simulink model "untitled1"  (R2025a)
settings: Solver=VariableStepAuto  StartTime=0.0  StopTime=5  RelTol=1e-3
libraries: spsControlledVoltageSourceLib x2, spsStepperMotorLib x1, spspowerguiLib x1
settings Model: Creator=One  LastModifiedBy=One

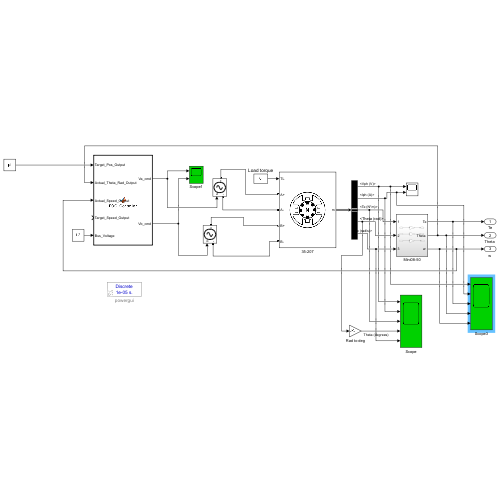
[thumbnail: Simulink's stored preview of the top-level diagram]
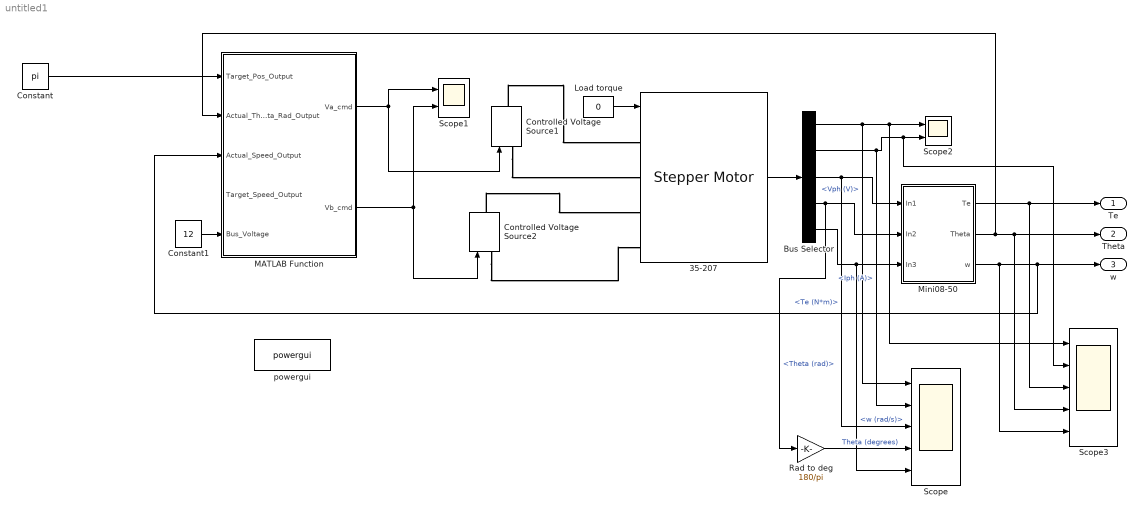
== system untitled1 ==
  35-207 : spsStepperMotorLib/Stepper Motor  MotorType=Permanent-magnet / Hybrid  NumberOfPhases_1=2  NumberOfPhases_2=3  PresetModel_1=<empty>  PresetModel_2=<empty>  L=5.44e-3  Lmax=10e-3  Lmin=2e-3  R=4.85  Step_angle=1.8  Psim=4.35e-3  Tdm=0.06  J=1e-6  B=1e-7*1000  w0=0  pos0=0  TsPowergui=0  TsBlock=-1
  Bus Selector : BusSelector  OutputSignals=Vph (V),Iph (A),Te (N*m),Theta (rad),w (rad/s)
  Constant : Constant  Value=pi
  Constant1 : Constant  Value=12
  Controlled Voltage Source1 : spsControlledVoltageSourceLib/Controlled Voltage Source  Initialize=on  Source_Type=AC  Amplitude=0  Phase=0  Frequency=0  Measurements=None
  Controlled Voltage Source2 : spsControlledVoltageSourceLib/Controlled Voltage Source  Initialize=on  Source_Type=AC  Amplitude=0  Phase=0  Frequency=0  Measurements=None
  Load torque : Constant  Value=0
  MATLAB Function : MATLAB Function  TreatAsAtomicUnit=on
  Mini08-50 : Subsystem
  Rad to deg : Gain  Gain=180/pi
  Scope : Scope  NumInputPorts=5
      settings: ActiveDisplayYMinimum=-13.428667964223356  ActiveDisplayYMaximum=11.64782499034316  DataLoggingVariableName=ScopeData2  DataLoggingSaveFormat=Array
  Scope1 : Scope  NumInputPorts=2
      settings: ActiveDisplayYMinimum=-30  ActiveDisplayYMaximum=30  DataLoggingSaveFormat=Array
  Scope2 : Scope  NumInputPorts=2
      settings: ActiveDisplayYMinimum=-30.084081407334793  ActiveDisplayYMaximum=16.419826459994084
  Scope3 : Scope  NumInputPorts=5
      settings: ActiveDisplayYMinimum=-13.428667964223356  ActiveDisplayYMaximum=11.64782499034316  DataLoggingVariableName=ScopeData3  DataLoggingSaveFormat=Array
  powergui : spspowerguiLib/powergui  SimulationMode=Discrete  SampleTime=1e-5  frequency=60  Iterations=50  frequencyindice=0  Pbase=100e6  ErrMax=1e-4  UnitsV=kV  UnitsW=MW  buscounter=0  FunctionMessages=off  echomessages=off  EnableUseOfTLC=off  CurrentSourceSwitches=off  DisableSnubberDevices=off  DisableRonSwitches=off  DisableVfSwitches=off  DisplayEquations=off  AutomaticDiscreteSolvers=off  SolverType=Tustin/Backward Euler (TBE)  Interpol=off  ExternalGateDelay=off  methode=off  Ts=0  x0status=blocks  SPID=off  SwTol=0  HookPort=off  NonlinearTolerance=1e-4  nMaxIteration=100  ContinueOnMaxIteration=off  RestoreLinks=warning  ResistiveCurrentMeasurement=off  Frange=[0:2:500]  Ylog=off  Xlog=on  ShowGrid=off  save=off  variable=ZData  structure=0  ZoomFFT=on  StartTime=0.0  cycles=1  DisplayStyle=1  fundamental=60  FreqAxis=off  MaxFrequency=1000  frequencyindicesteady=1  RmsSteady=1  display=off
  Te : Outport
  "Theta " : Outport  Port=2
  "w " : Outport  Port=3
  wires:
  Bus Selector/5 -> Scope/5, Mini08-50/3(In3)  "<w (rad/s)>"
  Constant1/1 -> MATLAB Function/5(Bus_Voltage)
  MATLAB Function/1(Va_cmd) -> Controlled Voltage Source1/1, Scope1/1
  Bus Selector/4 -> Rad to deg/1, Mini08-50/2(In2)  "<Theta (rad)>"
  Bus Selector/1 -> Scope/1, Scope3/1, Scope2/1  "<Vph (V)>"
  Mini08-50/3("w ") -> Scope3/5, MATLAB Function/3(Actual_Speed_Output), "w "/1
  35-207/1 -> Bus Selector/1
  Bus Selector/3 -> Scope/3, Mini08-50/1(In1)  "<Te (N*m)>"
  Bus Selector/2 -> Scope/2, Scope3/2, Scope2/2  "<Iph (A)>"
  Constant/1 -> MATLAB Function/1(Target_Pos_Output)
  Load torque/1 -> 35-207/1
  Mini08-50/2("Theta ") -> MATLAB Function/2(Actual_Theta_Rad_Output), Scope3/4, "Theta "/1
  MATLAB Function/2(Vb_cmd) -> Controlled Voltage Source2/1, Scope1/2
  Mini08-50/1(Te) -> Scope3/3, Te/1
  Rad to deg/1 -> Scope/4  "Theta (degrees)"
  connections:
  Controlled Voltage Source1/LConn1 -- 35-207/LConn2
  Controlled Voltage Source1/RConn1 -- 35-207/LConn1
  Controlled Voltage Source2/LConn1 -- 35-207/LConn4
  Controlled Voltage Source2/RConn1 -- 35-207/LConn3

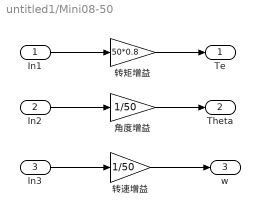
== system untitled1/Mini08-50 ==
  In1 : Inport
  In2 : Inport  Port=2
  In3 : Inport  Port=3
  角度增益 : Gain  Gain=1/50
  转矩增益 : Gain  Gain=50*0.8
  转速增益 : Gain  Gain=1/50
  Te : Outport
  "Theta " : Outport  Port=2
  "w " : Outport  Port=3
  wires:
  In3/1 -> 转速增益/1
  In1/1 -> 转矩增益/1
  转速增益/1 -> "w "/1
  转矩增益/1 -> Te/1
  角度增益/1 -> "Theta "/1
  In2/1 -> 角度增益/1

== matlab function untitled1/MATLAB Function ==
  data: Target_Pos_Output input; Va_cmd output; Actual_Theta_Rad_Output input; Actual_Speed_Output input; Target_Speed_Output input; Bus_Voltage input; Vb_cmd output
function [Va_cmd, Vb_cmd] = FOC_Controller(Target_Pos_Output, Actual_Theta_Rad_Output, Actual_Speed_Output, Target_Speed_Output, Bus_Voltage)
    % =========================================================================
    %  FOC 闭环控制器 (提升跟踪速度版) - 适配减速比50
    % 新增输入：Target_Speed_Output (输出轴目标速度，rad/s) —— 用于前馈补偿
    % =========================================================================
    
    % --- 1. 基础参数设置 ---
    PolePairs   = 50;     % 电机极对数
    Max_Current = 2.0;    % 电机最大允许电流 (A)
    GearRatio   = 50;     % 减速器减速比
    
    % [核心参数调优 - 提升响应速度的关键]
    Kp_pos = 50.0;        % 位置环 P (原8 → 大幅提升至25，根据震荡情况微调)
    Kv_pos = 0.8;         % 速度环 D (原0.25 → 同步提升，抑制P增大后的震荡)
    
    % [前馈参数 - 新增速度前馈]
    Ke = 0.08;            % 电机反电动势常数
    Kff_v = 1;          % 新增：速度前馈增益 (0~1之间，越大跟踪越快，过大易超调)
    
    Current_Gain = 5;   % 电流环增益 (原1.5 → 适当提升，加快电压响应)

    % --- 2. 输出轴 → 电机轴换算 ---
    Target_Pos_Motor = Target_Pos_Output * GearRatio;
    %Actual_Theta_Rad_Output = Actual_Theta_Deg_Output * (pi/180);
    Theta_mech_rad_Motor = Actual_Theta_Rad_Output * GearRatio;
    Actual_Speed_Motor = Actual_Speed_Output * GearRatio;
    Target_Speed_Motor = Target_Speed_Output * GearRatio; % 新增：目标速度换算到电机轴

    % --- 3. 电角度计算 ---
    Theta_elec = Theta_mech_rad_Motor * PolePairs;
    
    % --- 4. 控制律计算 (PD + 更大的P) ---
    Pos_Error = Target_Pos_Motor - Theta_mech_rad_Motor;
    I_target = Pos_Error * Kp_pos - Actual_Speed_Motor * Kv_pos; % 更大的P主导响应
    
    % 电流限幅
    if I_target > Max_Current, I_target = Max_Current;
    elseif I_target < -Max_Current, I_target = -Max_Current;
    end

    % --- 5. 坐标变换 ---
    Theta_foc = Theta_elec + (pi / 2); 
    I_alpha = I_target * cos(Theta_foc);
    I_beta  = I_target * sin(Theta_foc);
    
    % --- 6. 增强前馈补偿 (反电动势 + 速度前馈) ---
    % 1. 原有反电动势补偿 (基于实际速度)
    V_bemf_alpha = -Actual_Speed_Motor * Ke * sin(Theta_elec);
    V_bemf_beta  =  Actual_Speed_Motor * Ke * cos(Theta_elec);
    
    % 2. 新增：速度前馈补偿 (基于目标速度，提前驱动)
    % 将目标速度转换为Q轴电压，再投影到Alpha-Beta
    V_ff_q = Target_Speed_Motor * Kff_v; % 目标速度前馈电压
    V_ff_alpha = V_ff_q * cos(Theta_foc); % 投影到Alpha轴
    V_ff_beta  = V_ff_q * sin(Theta_foc); % 投影到Beta轴
    
    % --- 7. 最终输出计算 (PID + 反电动势 + 速度前馈) ---
    Va_raw = (I_alpha * Current_Gain) + V_bemf_alpha + V_ff_alpha;
    Vb_raw = (I_beta  * Current_Gain) + V_bemf_beta  + V_ff_beta;
    
    % --- 8. 电压限幅 ---
    if Va_raw > Bus_Voltage, Va_cmd = Bus_Voltage; 
    elseif Va_raw < -Bus_Voltage, Va_cmd = -Bus_Voltage;
    else, Va_cmd = Va_raw;
    end
    
    if Vb_raw > Bus_Voltage, Vb_cmd = Bus_Voltage;
    elseif Vb_raw < -Bus_Voltage, Vb_cmd = -Bus_Voltage;
    else, Vb_cmd = Vb_raw;
    end
    
end
